simulink model "maain"  (Simulink 7.5)
settings: Solver=ode45  StartTime=0.0  StopTime=0.1  RelTol=1e-3
undefined symbols (not defined in the file): DiscIntNeverNeededParam, Hydride, Metal, Nickel, Ts
libraries: elec_lib x216, powerlib x32, fl_lib x9, powerlib_extras x7, electricdrivelib x2, simulink x2, nesl_utility x2
(part 2 of 2)

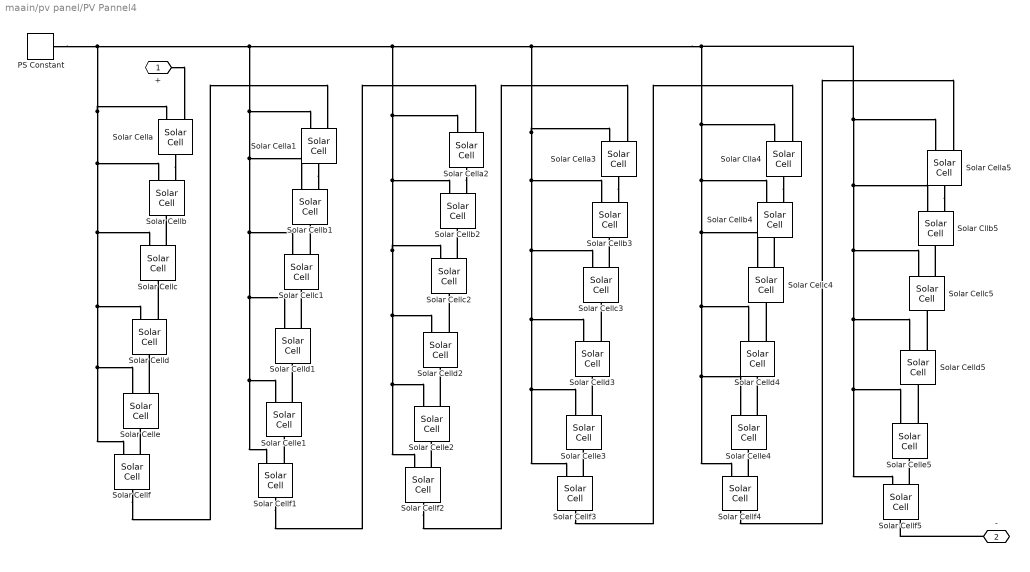
== system maain/pv panel/PV Pannel4 ==
  PS Constant : fl_lib/Physical Signals/Sources/PS Constant  DialogController=NetworkEngine.DynNeDlgSource  SystemSampleTime=-1  constant=687  LocalVarLogging=[]
  Solar Cella{,1..3,5} (5 alike) : elec_lib/Sources/Solar Cell  DialogController=NetworkEngine.DynNeDlgSource  SystemSampleTime=-1  prm=1  Isc=2.54 A  Voc=21.8 V  Is=1e-6 A  Is2=0 A  Iph=7.34 A  Ir0=1000 W/m^2  ec=1.6  N2=2  Rs=5.1e-3 Ohm  Rp=Inf Ohm  TIPH1=0.65e-3 1/K  EG=1.12 eV  TXIS1=3  TXIS2=3  TRS1=0  TRP1=0  TFIXED=25 C  Tmeas=25 C  LocalVarLogging=[]
  Solar Cellb{,1..4} (5 alike) : elec_lib/Sources/Solar Cell  DialogController=NetworkEngine.DynNeDlgSource  SystemSampleTime=-1  prm=1  Isc=2.54 A  Voc=21.8 V  Is=1e-6 A  Is2=0 A  Iph=7.34 A  Ir0=1000 W/m^2  ec=1.6  N2=2  Rs=5.1e-3 Ohm  Rp=Inf Ohm  TIPH1=0.65e-3 1/K  EG=1.12 eV  TXIS1=3  TXIS2=3  TRS1=0  TRP1=0  TFIXED=25 C  Tmeas=25 C  LocalVarLogging=[]
  Solar Cellc{,1..5} (6 alike) : elec_lib/Sources/Solar Cell  DialogController=NetworkEngine.DynNeDlgSource  SystemSampleTime=-1  prm=1  Isc=2.54 A  Voc=21.8 V  Is=1e-6 A  Is2=0 A  Iph=7.34 A  Ir0=1000 W/m^2  ec=1.6  N2=2  Rs=5.1e-3 Ohm  Rp=Inf Ohm  TIPH1=0.65e-3 1/K  EG=1.12 eV  TXIS1=3  TXIS2=3  TRS1=0  TRP1=0  TFIXED=25 C  Tmeas=25 C  LocalVarLogging=[]
  Solar Celld{,1..5} (6 alike) : elec_lib/Sources/Solar Cell  DialogController=NetworkEngine.DynNeDlgSource  SystemSampleTime=-1  prm=1  Isc=2.54 A  Voc=21.8 V  Is=1e-6 A  Is2=0 A  Iph=7.34 A  Ir0=1000 W/m^2  ec=1.6  N2=2  Rs=5.1e-3 Ohm  Rp=Inf Ohm  TIPH1=0.65e-3 1/K  EG=1.12 eV  TXIS1=3  TXIS2=3  TRS1=0  TRP1=0  TFIXED=25 C  Tmeas=25 C  LocalVarLogging=[]
  Solar Celle{,1..5} (6 alike) : elec_lib/Sources/Solar Cell  DialogController=NetworkEngine.DynNeDlgSource  SystemSampleTime=-1  prm=1  Isc=2.54 A  Voc=21.8 V  Is=1e-6 A  Is2=0 A  Iph=7.34 A  Ir0=1000 W/m^2  ec=1.6  N2=2  Rs=5.1e-3 Ohm  Rp=Inf Ohm  TIPH1=0.65e-3 1/K  EG=1.12 eV  TXIS1=3  TXIS2=3  TRS1=0  TRP1=0  TFIXED=25 C  Tmeas=25 C  LocalVarLogging=[]
  Solar Cellf{,1..5} (6 alike) : elec_lib/Sources/Solar Cell  DialogController=NetworkEngine.DynNeDlgSource  SystemSampleTime=-1  prm=1  Isc=2.54 A  Voc=21.8 V  Is=1e-6 A  Is2=0 A  Iph=7.34 A  Ir0=1000 W/m^2  ec=1.6  N2=2  Rs=5.1e-3 Ohm  Rp=Inf Ohm  TIPH1=0.65e-3 1/K  EG=1.12 eV  TXIS1=3  TXIS2=3  TRS1=0  TRP1=0  TFIXED=25 C  Tmeas=25 C  LocalVarLogging=[]
  Solar Clla4 : elec_lib/Sources/Solar Cell  DialogController=NetworkEngine.DynNeDlgSource  SystemSampleTime=-1  prm=1  Isc=2.54 A  Voc=21.8 V  Is=1e-6 A  Is2=0 A  Iph=7.34 A  Ir0=1000 W/m^2  ec=1.6  N2=2  Rs=5.1e-3 Ohm  Rp=Inf Ohm  TIPH1=0.65e-3 1/K  EG=1.12 eV  TXIS1=3  TXIS2=3  TRS1=0  TRP1=0  TFIXED=25 C  Tmeas=25 C  LocalVarLogging=[]
  Solar Cllb5 : elec_lib/Sources/Solar Cell  DialogController=NetworkEngine.DynNeDlgSource  SystemSampleTime=-1  prm=1  Isc=2.54 A  Voc=21.8 V  Is=1e-6 A  Is2=0 A  Iph=7.34 A  Ir0=1000 W/m^2  ec=1.6  N2=2  Rs=5.1e-3 Ohm  Rp=Inf Ohm  TIPH1=0.65e-3 1/K  EG=1.12 eV  TXIS1=3  TXIS2=3  TRS1=0  TRP1=0  TFIXED=25 C  Tmeas=25 C  LocalVarLogging=[]
  + : PMIOPort  Port=1  Side=Left
  - : PMIOPort  Port=2  Side=Left
  connections:
  -/RConn1 -- Solar Cellf5/RConn1
  +/RConn1 -- Solar Cella/LConn2
  Solar Cella3/LConn1 -- Solar Cellb3/LConn1 -- Solar Cellc3/LConn1 -- Solar Celld3/LConn1 -- Solar Celle3/LConn1 -- Solar Cellf3/LConn1 -- Solar Celle2/LConn1 -- Solar Cellf2/LConn1 -- Solar Celld2/LConn1 -- Solar Cellc2/LConn1 -- Solar Cellb2/LConn1 -- Solar Cella2/LConn1 -- Solar Cella1/LConn1 -- Solar Cellb1/LConn1 -- Solar Cellc1/LConn1 -- Solar Celld1/LConn1 -- Solar Celle1/LConn1 -- Solar Cellf1/LConn1 -- Solar Cella/LConn1 -- Solar Cellb/LConn1 -- Solar Cellc/LConn1 -- Solar Celld/LConn1 -- Solar Celle/LConn1 -- Solar Cellf/LConn1 -- PS Constant/RConn1 -- Solar Celle5/LConn1 -- Solar Cellf5/LConn1 -- Solar Celld5/LConn1 -- Solar Cellc5/LConn1 -- Solar Cllb5/LConn1 -- Solar Cella5/LConn1 -- Solar Clla4/LConn1 -- Solar Cellb4/LConn1 -- Solar Cellc4/LConn1 -- Solar Celld4/LConn1 -- Solar Celle4/LConn1 -- Solar Cellf4/LConn1
  Solar Cellf4/RConn1 -- Solar Cella5/LConn2
  Solar Cellf3/RConn1 -- Solar Clla4/LConn2
  Solar Cellf2/RConn1 -- Solar Cella3/LConn2
  Solar Cellf1/RConn1 -- Solar Cella2/LConn2
  Solar Cellf/RConn1 -- Solar Cella1/LConn2
  Solar Cellf5/LConn2 -- Solar Celle5/RConn1
  Solar Celle5/LConn2 -- Solar Celld5/RConn1
  Solar Celld5/LConn2 -- Solar Cellc5/RConn1
  Solar Cellc5/LConn2 -- Solar Cllb5/RConn1
  Solar Cella5/RConn1 -- Solar Cllb5/LConn2
  Solar Cellf4/LConn2 -- Solar Celle4/RConn1
  Solar Celle4/LConn2 -- Solar Celld4/RConn1
  Solar Celld4/LConn2 -- Solar Cellc4/RConn1
  Solar Cellc4/LConn2 -- Solar Cellb4/RConn1
  Solar Clla4/RConn1 -- Solar Cellb4/LConn2
  Solar Cellf3/LConn2 -- Solar Celle3/RConn1
  Solar Celle3/LConn2 -- Solar Celld3/RConn1
  Solar Celld3/LConn2 -- Solar Cellc3/RConn1
  Solar Cellc3/LConn2 -- Solar Cellb3/RConn1
  Solar Cella3/RConn1 -- Solar Cellb3/LConn2
  Solar Cellf2/LConn2 -- Solar Celle2/RConn1
  Solar Celle2/LConn2 -- Solar Celld2/RConn1
  Solar Celld2/LConn2 -- Solar Cellc2/RConn1
  Solar Cellc2/LConn2 -- Solar Cellb2/RConn1
  Solar Cella2/RConn1 -- Solar Cellb2/LConn2
  Solar Cellf1/LConn2 -- Solar Celle1/RConn1
  Solar Celle1/LConn2 -- Solar Celld1/RConn1
  Solar Celld1/LConn2 -- Solar Cellc1/RConn1
  Solar Cellc1/LConn2 -- Solar Cellb1/RConn1
  Solar Cella1/RConn1 -- Solar Cellb1/LConn2
  Solar Cellf/LConn2 -- Solar Celle/RConn1
  Solar Celle/LConn2 -- Solar Celld/RConn1
  Solar Celld/LConn2 -- Solar Cellc/RConn1
  Solar Cellc/LConn2 -- Solar Cellb/RConn1
  Solar Cella/RConn1 -- Solar Cellb/LConn2

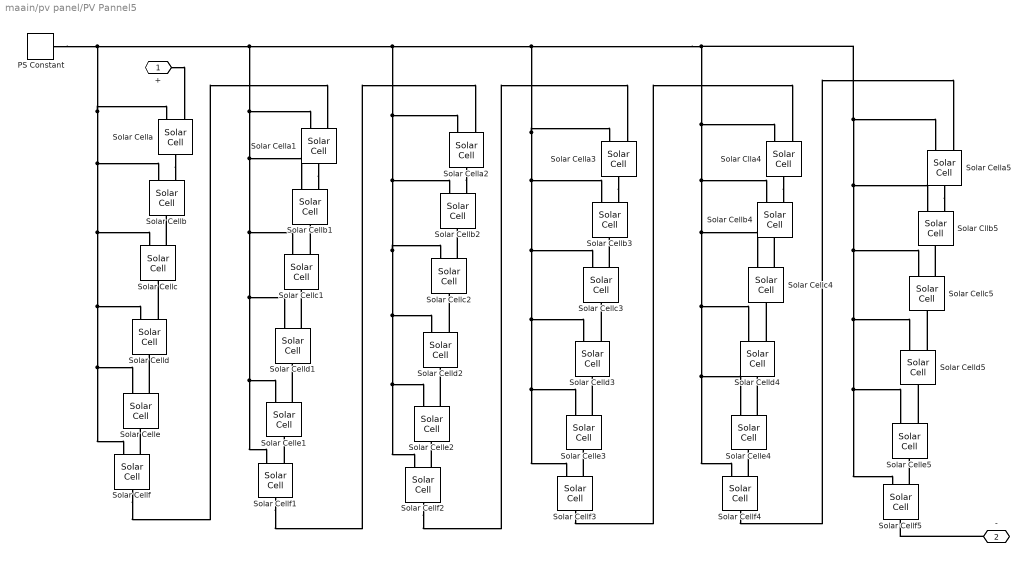
== system maain/pv panel/PV Pannel5 ==
  PS Constant : fl_lib/Physical Signals/Sources/PS Constant  DialogController=NetworkEngine.DynNeDlgSource  SystemSampleTime=-1  constant=687  LocalVarLogging=[]
  Solar Cella{,1..3,5} (5 alike) : elec_lib/Sources/Solar Cell  DialogController=NetworkEngine.DynNeDlgSource  SystemSampleTime=-1  prm=1  Isc=2.54 A  Voc=21.8 V  Is=1e-6 A  Is2=0 A  Iph=7.34 A  Ir0=1000 W/m^2  ec=1.6  N2=2  Rs=5.1e-3 Ohm  Rp=Inf Ohm  TIPH1=0.65e-3 1/K  EG=1.12 eV  TXIS1=3  TXIS2=3  TRS1=0  TRP1=0  TFIXED=25 C  Tmeas=25 C  LocalVarLogging=[]
  Solar Cellb{,1..4} (5 alike) : elec_lib/Sources/Solar Cell  DialogController=NetworkEngine.DynNeDlgSource  SystemSampleTime=-1  prm=1  Isc=2.54 A  Voc=21.8 V  Is=1e-6 A  Is2=0 A  Iph=7.34 A  Ir0=1000 W/m^2  ec=1.6  N2=2  Rs=5.1e-3 Ohm  Rp=Inf Ohm  TIPH1=0.65e-3 1/K  EG=1.12 eV  TXIS1=3  TXIS2=3  TRS1=0  TRP1=0  TFIXED=25 C  Tmeas=25 C  LocalVarLogging=[]
  Solar Cellc{,1..5} (6 alike) : elec_lib/Sources/Solar Cell  DialogController=NetworkEngine.DynNeDlgSource  SystemSampleTime=-1  prm=1  Isc=2.54 A  Voc=21.8 V  Is=1e-6 A  Is2=0 A  Iph=7.34 A  Ir0=1000 W/m^2  ec=1.6  N2=2  Rs=5.1e-3 Ohm  Rp=Inf Ohm  TIPH1=0.65e-3 1/K  EG=1.12 eV  TXIS1=3  TXIS2=3  TRS1=0  TRP1=0  TFIXED=25 C  Tmeas=25 C  LocalVarLogging=[]
  Solar Celld{,1..5} (6 alike) : elec_lib/Sources/Solar Cell  DialogController=NetworkEngine.DynNeDlgSource  SystemSampleTime=-1  prm=1  Isc=2.54 A  Voc=21.8 V  Is=1e-6 A  Is2=0 A  Iph=7.34 A  Ir0=1000 W/m^2  ec=1.6  N2=2  Rs=5.1e-3 Ohm  Rp=Inf Ohm  TIPH1=0.65e-3 1/K  EG=1.12 eV  TXIS1=3  TXIS2=3  TRS1=0  TRP1=0  TFIXED=25 C  Tmeas=25 C  LocalVarLogging=[]
  Solar Celle{,1..5} (6 alike) : elec_lib/Sources/Solar Cell  DialogController=NetworkEngine.DynNeDlgSource  SystemSampleTime=-1  prm=1  Isc=2.54 A  Voc=21.8 V  Is=1e-6 A  Is2=0 A  Iph=7.34 A  Ir0=1000 W/m^2  ec=1.6  N2=2  Rs=5.1e-3 Ohm  Rp=Inf Ohm  TIPH1=0.65e-3 1/K  EG=1.12 eV  TXIS1=3  TXIS2=3  TRS1=0  TRP1=0  TFIXED=25 C  Tmeas=25 C  LocalVarLogging=[]
  Solar Cellf{,1..5} (6 alike) : elec_lib/Sources/Solar Cell  DialogController=NetworkEngine.DynNeDlgSource  SystemSampleTime=-1  prm=1  Isc=2.54 A  Voc=21.8 V  Is=1e-6 A  Is2=0 A  Iph=7.34 A  Ir0=1000 W/m^2  ec=1.6  N2=2  Rs=5.1e-3 Ohm  Rp=Inf Ohm  TIPH1=0.65e-3 1/K  EG=1.12 eV  TXIS1=3  TXIS2=3  TRS1=0  TRP1=0  TFIXED=25 C  Tmeas=25 C  LocalVarLogging=[]
  Solar Clla4 : elec_lib/Sources/Solar Cell  DialogController=NetworkEngine.DynNeDlgSource  SystemSampleTime=-1  prm=1  Isc=2.54 A  Voc=21.8 V  Is=1e-6 A  Is2=0 A  Iph=7.34 A  Ir0=1000 W/m^2  ec=1.6  N2=2  Rs=5.1e-3 Ohm  Rp=Inf Ohm  TIPH1=0.65e-3 1/K  EG=1.12 eV  TXIS1=3  TXIS2=3  TRS1=0  TRP1=0  TFIXED=25 C  Tmeas=25 C  LocalVarLogging=[]
  Solar Cllb5 : elec_lib/Sources/Solar Cell  DialogController=NetworkEngine.DynNeDlgSource  SystemSampleTime=-1  prm=1  Isc=2.54 A  Voc=21.8 V  Is=1e-6 A  Is2=0 A  Iph=7.34 A  Ir0=1000 W/m^2  ec=1.6  N2=2  Rs=5.1e-3 Ohm  Rp=Inf Ohm  TIPH1=0.65e-3 1/K  EG=1.12 eV  TXIS1=3  TXIS2=3  TRS1=0  TRP1=0  TFIXED=25 C  Tmeas=25 C  LocalVarLogging=[]
  + : PMIOPort  Port=1  Side=Left
  - : PMIOPort  Port=2  Side=Left
  connections:
  -/RConn1 -- Solar Cellf5/RConn1
  +/RConn1 -- Solar Cella/LConn2
  Solar Cella3/LConn1 -- Solar Cellb3/LConn1 -- Solar Cellc3/LConn1 -- Solar Celld3/LConn1 -- Solar Celle3/LConn1 -- Solar Cellf3/LConn1 -- Solar Celle2/LConn1 -- Solar Cellf2/LConn1 -- Solar Celld2/LConn1 -- Solar Cellc2/LConn1 -- Solar Cellb2/LConn1 -- Solar Cella2/LConn1 -- Solar Cella1/LConn1 -- Solar Cellb1/LConn1 -- Solar Cellc1/LConn1 -- Solar Celld1/LConn1 -- Solar Celle1/LConn1 -- Solar Cellf1/LConn1 -- Solar Cella/LConn1 -- Solar Cellb/LConn1 -- Solar Cellc/LConn1 -- Solar Celld/LConn1 -- Solar Celle/LConn1 -- Solar Cellf/LConn1 -- PS Constant/RConn1 -- Solar Celle5/LConn1 -- Solar Cellf5/LConn1 -- Solar Celld5/LConn1 -- Solar Cellc5/LConn1 -- Solar Cllb5/LConn1 -- Solar Cella5/LConn1 -- Solar Clla4/LConn1 -- Solar Cellb4/LConn1 -- Solar Cellc4/LConn1 -- Solar Celld4/LConn1 -- Solar Celle4/LConn1 -- Solar Cellf4/LConn1
  Solar Cellf4/RConn1 -- Solar Cella5/LConn2
  Solar Cellf3/RConn1 -- Solar Clla4/LConn2
  Solar Cellf2/RConn1 -- Solar Cella3/LConn2
  Solar Cellf1/RConn1 -- Solar Cella2/LConn2
  Solar Cellf/RConn1 -- Solar Cella1/LConn2
  Solar Cellf5/LConn2 -- Solar Celle5/RConn1
  Solar Celle5/LConn2 -- Solar Celld5/RConn1
  Solar Celld5/LConn2 -- Solar Cellc5/RConn1
  Solar Cellc5/LConn2 -- Solar Cllb5/RConn1
  Solar Cella5/RConn1 -- Solar Cllb5/LConn2
  Solar Cellf4/LConn2 -- Solar Celle4/RConn1
  Solar Celle4/LConn2 -- Solar Celld4/RConn1
  Solar Celld4/LConn2 -- Solar Cellc4/RConn1
  Solar Cellc4/LConn2 -- Solar Cellb4/RConn1
  Solar Clla4/RConn1 -- Solar Cellb4/LConn2
  Solar Cellf3/LConn2 -- Solar Celle3/RConn1
  Solar Celle3/LConn2 -- Solar Celld3/RConn1
  Solar Celld3/LConn2 -- Solar Cellc3/RConn1
  Solar Cellc3/LConn2 -- Solar Cellb3/RConn1
  Solar Cella3/RConn1 -- Solar Cellb3/LConn2
  Solar Cellf2/LConn2 -- Solar Celle2/RConn1
  Solar Celle2/LConn2 -- Solar Celld2/RConn1
  Solar Celld2/LConn2 -- Solar Cellc2/RConn1
  Solar Cellc2/LConn2 -- Solar Cellb2/RConn1
  Solar Cella2/RConn1 -- Solar Cellb2/LConn2
  Solar Cellf1/LConn2 -- Solar Celle1/RConn1
  Solar Celle1/LConn2 -- Solar Celld1/RConn1
  Solar Celld1/LConn2 -- Solar Cellc1/RConn1
  Solar Cellc1/LConn2 -- Solar Cellb1/RConn1
  Solar Cella1/RConn1 -- Solar Cellb1/LConn2
  Solar Cellf/LConn2 -- Solar Celle/RConn1
  Solar Celle/LConn2 -- Solar Celld/RConn1
  Solar Celld/LConn2 -- Solar Cellc/RConn1
  Solar Cellc/LConn2 -- Solar Cellb/RConn1
  Solar Cella/RConn1 -- Solar Cellb/LConn2

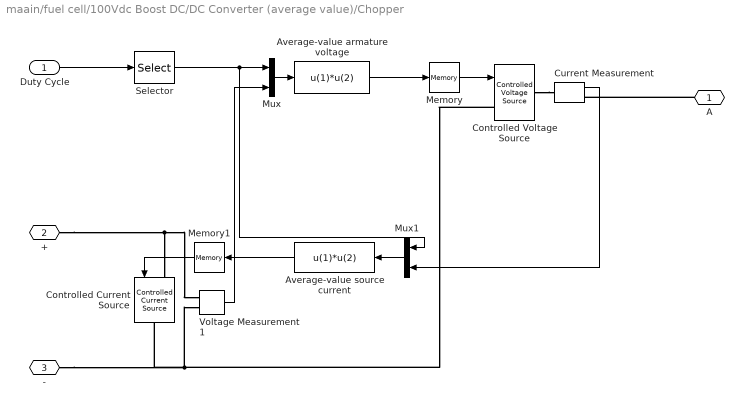
== system maain/fuel cell/100Vdc Boost DC/DC Converter (average value)/Chopper ==
  Duty Cycle : Inport  OutDataType=sfix(16)  OutScaling=2^0
  Average-value armature voltage : Fcn  Expr=u(1)*u(2)
  Average-value source current : Fcn  Expr=u(1)*u(2)
  Controlled Current Source : powerlib/Electrical Sources/Controlled Current Source  DialogController=POWERSYS.PowerSysDialog  SystemSampleTime=-1  Initialize=on  Source_Type=AC  Amplitude=0  Phase=0  Frequency=0  Measurements=None
  Controlled Voltage Source : powerlib/Electrical Sources/Controlled Voltage Source  DialogController=POWERSYS.PowerSysDialog  SystemSampleTime=-1  Initialize=on  Source_Type=AC  Amplitude=0  Phase=0  Frequency=0  Measurements=None
  Current Measurement : powerlib/Measurements/Current Measurement  Tag=PoWeRsYsTeMmEaSuReMeNt  DialogController=POWERSYS.PowerSysDialog  SystemSampleTime=-1  PhasorSimulation=off  OutputType=Magnitude  PSBequivalent=0
  Memory : Memory
  Memory1 : Memory
  Mux : Mux  Inputs=2
  Mux1 : Mux  Inputs=2
  Selector : Selector  InputPortWidth=2  IndexOptions=Index vector (dialog)  Indices=[1]  OutputSizes=1
  Voltage Measurement1 : powerlib/Measurements/Voltage Measurement  Tag=PoWeRsYsTeMmEaSuReMeNt  DialogController=POWERSYS.PowerSysDialog  SystemSampleTime=-1  PhasorSimulation=off  OutputType=Magnitude  PSBequivalent=0
  A : PMIOPort  Port=1  Side=Right
  + : PMIOPort  Port=2  Side=Left
  - : PMIOPort  Port=3  Side=Left
  wires:
  Selector/1 -> Mux1/1, Mux/1
  Memory1/1 -> Controlled Current Source/1
  Average-value source current/1 -> Memory1/1
  Current Measurement/1 -> Mux1/2
  Mux1/1 -> Average-value source current/1
  Duty Cycle/1 -> Selector/1
  Voltage Measurement1/1 -> Mux/2
  Mux/1 -> Average-value armature voltage/1
  Average-value armature voltage/1 -> Memory/1
  Memory/1 -> Controlled Voltage Source/1
  connections:
  A/RConn1 -- Current Measurement/RConn1
  Controlled Voltage Source/RConn1 -- Current Measurement/LConn1
  +/RConn1 -- Voltage Measurement1/LConn1 -- Controlled Current Source/LConn1
  Controlled Voltage Source/LConn1 -- -/RConn1 -- Controlled Current Source/RConn1 -- Voltage Measurement1/LConn2

== system maain/fuel cell/100Vdc Boost DC/DC Converter (average value)/Current controller DISCRETE1 ==
  UBus : Inport  OutDataType=sfix(16)  OutScaling=2^0
  Uref : Inport  Port=2  OutDataType=sfix(16)  OutScaling=2^0
  Ctrl sat. : Saturate  UpperLimit=0.95  LowerLimit=-0.95  OutDataType=sfix(16)  OutScaling=2^0
  Discrete-Time Integrator : DiscreteIntegrator  IntegratorMethod=Integration: Trapezoidal  SampleTime=Ts  OutDataType=sfix(16)  OutScaling=2^0  LimitOutput=on  UpperSaturationLimit=0.95  LowerSaturationLimit=-0.95  ICPrevOutput=DiscIntNeverNeededParam  ICPrevScaledInput=DiscIntNeverNeededParam
  Integral gain : Gain  Gain=Ki  ParameterDataType=sfix(16)  ParameterScaling=2^0  OutDataType=sfix(16)  OutScaling=2^0  SaturateOnIntegerOverflow=on  OutDataTypeStr=Inherit: Same as input  ParamDataTypeStr=Inherit: Same as input
  Proportional gain : Gain  Gain=Kp  ParameterDataType=sfix(16)  ParameterScaling=2^0  OutDataType=sfix(16)  OutScaling=2^0  SaturateOnIntegerOverflow=on  OutDataTypeStr=Inherit: Same as input  ParamDataTypeStr=Inherit: Same as input
  Sum1 : Sum  Inputs=+-  OutDataType=sfix(16)  OutScaling=2^0  SaturateOnIntegerOverflow=on  InputSameDT=on  OutDataTypeStr=Inherit: Same as first input
  Sum2 : Sum  OutDataType=sfix(16)  OutScaling=2^0  SaturateOnIntegerOverflow=on  InputSameDT=on  OutDataTypeStr=Inherit: Same as first input
  Ec : Outport  OutDataType=sfix(16)  OutScaling=2^0  InitialOutput=0
  wires:
  Ctrl sat./1 -> Ec/1
  Sum2/1 -> Ctrl sat./1
  Discrete-Time Integrator/1 -> Sum2/2
  Uref/1 -> Sum1/2
  UBus/1 -> Sum1/1
  Sum1/1 -> Proportional gain/1, Integral gain/1
  Integral gain/1 -> Discrete-Time Integrator/1
  Proportional gain/1 -> Sum2/1

== system maain/fuel cell/100Vdc Boost DC/DC Converter (average value)/Duty Cycles ==
  Ec : Inport  OutDataType=sfix(16)  OutScaling=2^0
  Add : Sum  Inputs=+-  OutDataType=sfix(16)  OutScaling=2^-10
  Bus Creator2 : BusCreator  Inputs=2
  Constant : Constant  OutDataType=sfix(16)  OutScaling=2^0
  Duty Cycle : Fcn  Expr=0.5*(u[1]+1)
  dc : Outport  OutDataType=sfix(16)  OutScaling=2^0
  wires:
  Bus Creator2/1 -> dc/1
  Ec/1 -> Duty Cycle/1
  Constant/1 -> Add/1
  Add/1 -> Bus Creator2/2  "IGBT 2"
  Duty Cycle/1 -> Bus Creator2/1, Add/2  "IGBT I"
